simulink model "Lab3"  (R2023a)
settings: Solver=ode45  StartTime=0.0  StopTime=100  RelTol=1e-3
StopFcn:
  | % figure
  | % plot(20*log10(abs(fft(filter_out))));
undefined symbols (not defined in the file): xc7k325tfbg676
libraries: hdlBasic x35, vmcUtilities x1, dspsrcs4 x1
settings Model: Creator=scaffee  LastModifiedBy=robg
settings SolverCC: AlgebraicLoopSolver=TrustRegion
settings DataIOCC: LimitDataPoints=on  SaveFormat=Array  SignalLoggingSaveFormat=ModelDataLogs  ReturnWorkspaceOutputs=off
settings OptimizationCC: BlockReduction=off  BooleanDataType=off  LifeSpan=inf
settings DebuggingCC: SaveWithParameterizedLinksMsg=none  UnderspecifiedInitializationDetection=Classic  MergeDetectMultiDrivingBlocksExec=none  SignalResolutionControl=TryResolveAllWithWarning  MultiTaskDSMMsg=warning  MultiTaskCondExecSysMsg=none  UnconnectedInputMsg=warning  UnconnectedOutputMsg=warning  UnconnectedLineMsg=warning  AllowSymbolicDim=off  StateNameClashWarn=warning  SFUnexpectedBacktrackingDiag=warning  SFNoUnconditionalDefaultTransitionDiag=warning  ArithmeticOperatorsInVariantConditions=warning
settings HardwareCC: ProdBitPerPointer=32  ProdBitPerSizeT=32  ProdBitPerPtrDiffT=32  ProdLargestAtomicFloat=None  ProdIntDivRoundTo=Undefined  ProdEndianess=Unspecified  ProdWordSize=32  ProdHWDeviceType=32-bit Generic  TargetUnknown=on
settings ModelReferenceCC: EnableRefExpFcnMdlSchedulingChecks=on  PropagateSignalLabelsOutOfModel=off
settings SFSimCC: SimUseLocalCustomCode=off  CustomCodeUndefinedFunction=UseInterfaceOnly
settings RTWCC: RTWUseLocalCustomCode=off  DLArmComputeVersion=19.05
settings CodeAppCC: StateflowObjectComments=on
settings GRTTargetCC: TargetLangStandard=C89/C90 (ANSI)
settings ConfigComp: CovMetricSettings=dw  CovSaveCumulativeToWorkspaceVar=on  CovSaveSingleToWorkspaceVar=on  CovExternalEMLEnable=off

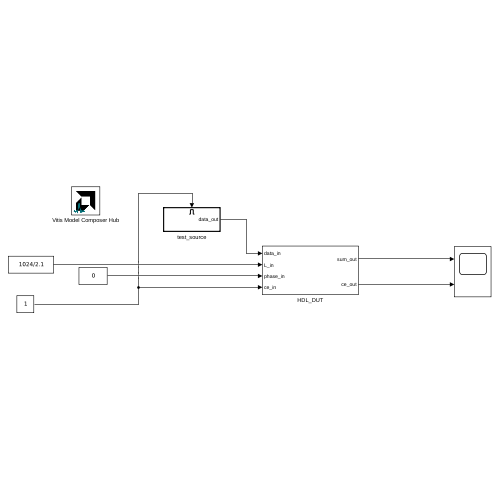
[thumbnail: Simulink's stored preview of the top-level diagram]
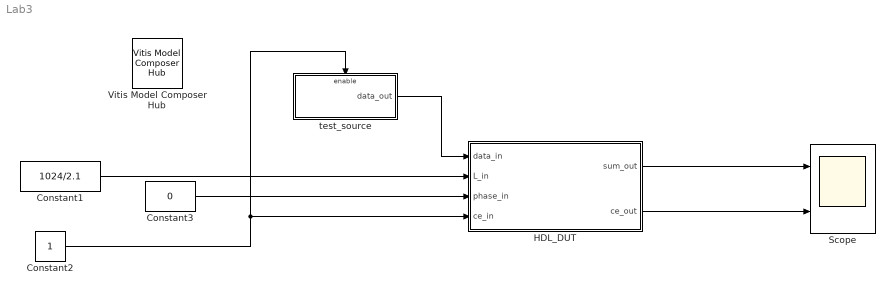
== system Lab3 ==
  Constant1 : Constant  Value=1024/2.1
  Constant2 : Constant
  Constant3 : Constant  Value=0
  HDL_DUT : Subsystem
  Scope : Scope  NumInputPorts=2
  Vitis Model Composer Hub : vmcUtilities/Vitis Model Composer Hub  Tag=genX  CodeGeneration=off  SubsystemName=HDL_DUT  StartColumn=1  NumberOfColumns=1  TargetDirectory=./code  exportDesign=off  analyzeDesign=off  validateDesignOnHw=off  ExportType=System Generator  IpVendor=xilinx.com  IpLibrary=hls  IpVersion=1.0  IpHWLanguage=Verilog  AieCompilerOptions={}  AieSimulatorOptions={}  CreateTestbench=off  TestbenchStackSize=10  RunRtlSim=off  RunCSim=off  RunAieSim=off  AieSimTimeout=50000  RunAieSimProfiling=off  LaunchVitisAnalyzer=off  PlotOutput=off  RunX86Sim=off  X86SimTimeout=10  GenHwImage=off  GenLibadfXo=on  GenHwValidationCode=off  PlatformType=Not Specified  HwSystemType=Baremetal  HwValidationTarget=hw  ProjDevice=xc7k325tfbg676-3  ProjDevicePart=xc7k325tfbg676-3  SamplePeriod=-1  ClockFrequency=200  DataPathParallelism=1  xilinxfamily=kintex7  part=xc7k325t  speed=-3  package=fbg676  directory=./netlist/ip/HDL_DUT/src  testbench=off  incr_netlist=off  synthesis_tool=Vivado  clock_wrapper=Clock Enables  dbl_ovrd=According to Block Masks  dcm_input_clock_period=10  sysclk_period=4  simulink_period=1  eval_field=0  LogFileName=''  NThreads=4
  test_source : Subsystem  TreatAsAtomicUnit=on
  wires:
  Constant2/1 -> HDL_DUT/4(ce_in), test_source/Enable
  test_source/1(data_out) -> HDL_DUT/1(data_in)
  Constant1/1 -> HDL_DUT/2(L_in)
  Constant3/1 -> HDL_DUT/3(phase_in)
  HDL_DUT/1(sum_out) -> Scope/1
  HDL_DUT/2(ce_out) -> Scope/2

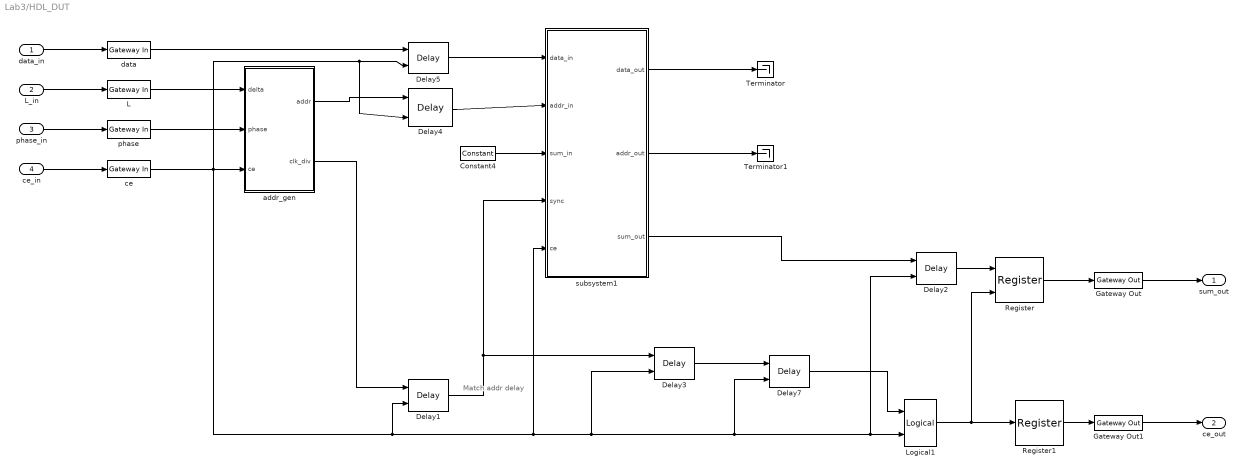
== system Lab3/HDL_DUT ==
  note: Match addr delay
  data_in : Inport
  L_in : Inport  Port=2
  phase_in : Inport  Port=3
  ce_in : Inport  Port=4
  Constant4 : hdlBasic/Constant  const=0  gui_display_data_type=Fixed-point  arith_type=Signed (2's comp)  n_bits=48  bin_pt=34  preci_type=Single  exp_width=8  frac_width=24  explicit_period=off  period=1  XmcBlockStatus=1  maskContainerNames=tabcontainer1  block_type=constant  block_config=sysgen:Constant_config
  Delay1 : hdlBasic/Delay  rst=off  en=on  latency=2  reg_retiming=on  XmcBlockStatus=1  maskContainerNames=group1  block_type=delay  block_config=sysgen:Delay_config
  Delay2 : hdlBasic/Delay  rst=off  en=on  latency=1  reg_retiming=on  XmcBlockStatus=1  maskContainerNames=group1  block_type=delay  block_config=sysgen:Delay_config
  Delay3 : hdlBasic/Delay  rst=off  en=on  latency=4  reg_retiming=on  XmcBlockStatus=1  maskContainerNames=group1  block_type=delay  block_config=sysgen:Delay_config
  Delay4 : hdlBasic/Delay  rst=off  en=on  latency=2  reg_retiming=on  XmcBlockStatus=1  maskContainerNames=group1  block_type=delay  block_config=sysgen:Delay_config
  Delay5 : hdlBasic/Delay  rst=off  en=on  latency=2  reg_retiming=on  XmcBlockStatus=1  maskContainerNames=group1  block_type=delay  block_config=sysgen:Delay_config
  Delay7 : hdlBasic/Delay  rst=off  en=on  latency=1  reg_retiming=on  XmcBlockStatus=1  maskContainerNames=group1  block_type=delay  block_config=sysgen:Delay_config
  Gateway Out : hdlBasic/Gateway Out  inherit_from_input=off  hdl_port=on  rows=1  columns=1  UseAsDAC=off  DACChannel='1'  interface=None  automatic_assignment=on  address_offset=hex2dec('00')  intf_name=''  intf_description=''  timing_constraint=None  locs_specified=off  LOCs={}  io_standard={}  XmcBlockStatus=1  maskContainerNames=group4  block_type=gatewayout  block_config=sysgen:gateway_out_config  block_width_w=590  block_height_w=620  block_width=620  block_height=750
  Gateway Out1 : hdlBasic/Gateway Out  inherit_from_input=off  hdl_port=on  rows=1  columns=1  UseAsDAC=off  DACChannel='1'  interface=None  automatic_assignment=on  address_offset=hex2dec('00')  intf_name=''  intf_description=''  timing_constraint=None  locs_specified=off  LOCs={}  io_standard={}  XmcBlockStatus=1  maskContainerNames=group4  block_type=gatewayout  block_config=sysgen:gateway_out_config  block_width_w=590  block_height_w=620  block_width=620  block_height=750
  L : hdlBasic/Gateway In  gui_display_data_type=Fixed-point  arith_type=Unsigned  n_bits=32  bin_pt=21  preci_type=Single  exp_width=8  frac_width=24  rows=1  columns=1  quantization="Round  (unbiased: +/- Inf)"  overflow=Saturate  period=1  UseAsADC=off  ADCChannel='1'  interface=None  automatic_assignment=on  address_offset=hex2dec('00')  intf_name=''  intf_description=''  default_value=0  timing_constraint=None  locs_specified=off  LOCs={}  io_standard={}  inherit_from_input=off  hdl_port=on  XmcBlockStatus=1  maskContainerNames=group4  block_type=gatewayin  block_config=sysgen:gateway_in_config  block_width_w=590  block_height_w=620  block_width=640  block_height=850
  Logical1 : hdlBasic/Logical  logical_function=AND  inputs=2  en=off  latency=0  precision=Full  arith_type=Unsigned  n_bits=8  bin_pt=2  align_bp=on  overflow=[]  quantization=[]  XmcBlockStatus=1  maskContainerNames=tabcontainer1  block_type=logical  block_config=sysgen:Logical_config
  Register : hdlBasic/Register  init=0  rst=off  en=on  XmcBlockStatus=1  maskContainerNames=tabcontainer1  block_type=register  block_config=sysgen:Register_config
  Register1 : hdlBasic/Register  init=0  rst=off  en=off  XmcBlockStatus=1  maskContainerNames=tabcontainer1  block_type=register  block_config=sysgen:Register_config
  Terminator : Terminator
  Terminator1 : Terminator
  addr_gen : Subsystem
  ce : hdlBasic/Gateway In  gui_display_data_type=Boolean  arith_type=Boolean  n_bits=8  bin_pt=0  preci_type=Single  exp_width=8  frac_width=24  rows=1  columns=1  quantization="Round  (unbiased: +/- Inf)"  overflow=Saturate  period=1  UseAsADC=off  ADCChannel='1'  interface=None  automatic_assignment=on  address_offset=hex2dec('00')  intf_name=''  intf_description=''  default_value=0  timing_constraint=None  locs_specified=off  LOCs={}  io_standard={}  inherit_from_input=off  hdl_port=on  XmcBlockStatus=1  maskContainerNames=group4  block_type=gatewayin  block_config=sysgen:gateway_in_config  block_width_w=590  block_height_w=620  block_width=640  block_height=850
  data : hdlBasic/Gateway In  gui_display_data_type=Fixed-point  arith_type=Signed (2's comp)  n_bits=18  bin_pt=17  preci_type=Single  exp_width=8  frac_width=24  rows=1  columns=1  quantization="Round  (unbiased: +/- Inf)"  overflow=Saturate  period=1  UseAsADC=off  ADCChannel='1'  interface=None  automatic_assignment=on  address_offset=hex2dec('00')  intf_name=''  intf_description=''  default_value=0  timing_constraint=None  locs_specified=off  LOCs={}  io_standard={}  inherit_from_input=off  hdl_port=on  XmcBlockStatus=1  maskContainerNames=group4  block_type=gatewayin  block_config=sysgen:gateway_in_config  block_width_w=590  block_height_w=620  block_width=640  block_height=850
  phase : hdlBasic/Gateway In  gui_display_data_type=Fixed-point  arith_type=Unsigned  n_bits=10  bin_pt=0  preci_type=Single  exp_width=8  frac_width=24  rows=1  columns=1  quantization="Round  (unbiased: +/- Inf)"  overflow=Saturate  period=1  UseAsADC=off  ADCChannel='1'  interface=None  automatic_assignment=on  address_offset=hex2dec('00')  intf_name=''  intf_description=''  default_value=0  timing_constraint=None  locs_specified=off  LOCs={}  io_standard={}  inherit_from_input=off  hdl_port=on  XmcBlockStatus=1  maskContainerNames=group4  block_type=gatewayin  block_config=sysgen:gateway_in_config  block_width_w=590  block_height_w=620  block_width=640  block_height=850
  subsystem1 : Subsystem  mask{hhpoly1=8}
      mask prompts: hhpoly1 "Filter coefficients column?"
  sum_out : Outport
  ce_out : Outport  Port=2
  wires:
  addr_gen/1(addr) -> Delay4/1
  subsystem1/3(sum_out) -> Delay2/1
  Register1/1 -> Gateway Out1/1
  Delay2/1 -> Register/1
  Delay4/1 -> subsystem1/2(addr_in)
  Gateway Out/1 -> sum_out/1
  Delay5/1 -> subsystem1/1(data_in)
  addr_gen/2(clk_div) -> Delay1/1
  Gateway Out1/1 -> ce_out/1
  phase/1 -> addr_gen/2(phase)
  ce_in/1 -> ce/1
  Delay7/1 -> Logical1/1
  data/1 -> Delay5/1
  L_in/1 -> L/1
  phase_in/1 -> phase/1
  Logical1/1 -> Register/2, Register1/1
  Constant4/1 -> subsystem1/3(sum_in)
  subsystem1/2(addr_out) -> Terminator1/1
  subsystem1/1(data_out) -> Terminator/1
  Delay1/1 -> subsystem1/4(sync), Delay3/1
  Register/1 -> Gateway Out/1
  ce/1 -> Delay4/2, Delay5/2, addr_gen/3(ce), Delay1/2, subsystem1/5(ce), Delay3/2, Delay7/2, Delay2/2, Logical1/2
  data_in/1 -> data/1
  L/1 -> addr_gen/1(delta)
  Delay3/1 -> Delay7/1

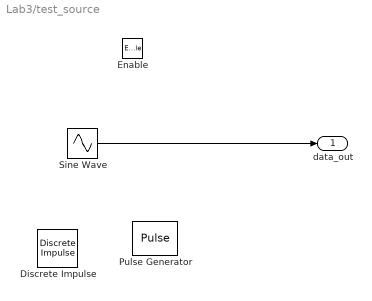
== system Lab3/test_source ==
  Enable : EnablePort
  Discrete Impulse : dspsrcs4/Discrete  Impulse  Delay=101  SampleTime=1  FrameSample=1  OutputFrames=on  dataType=double  isSigned=on  wordLen=16  udDataType=sfix(16)  fracBitsMode=Best precision  numFracBits=15  OutDataTypeStr=double  LastOutDataTypeStr=double
  Pulse Generator : DiscretePulseGenerator  Period=2048  PulseWidth=512
  Sine Wave : Sin  SineType=Sample based  Samples=3*1000  SampleTime=1
  data_out : Outport  VectorParamsAs1DForOutWhenUnconnected=off
  wires:
  Sine Wave/1 -> data_out/1

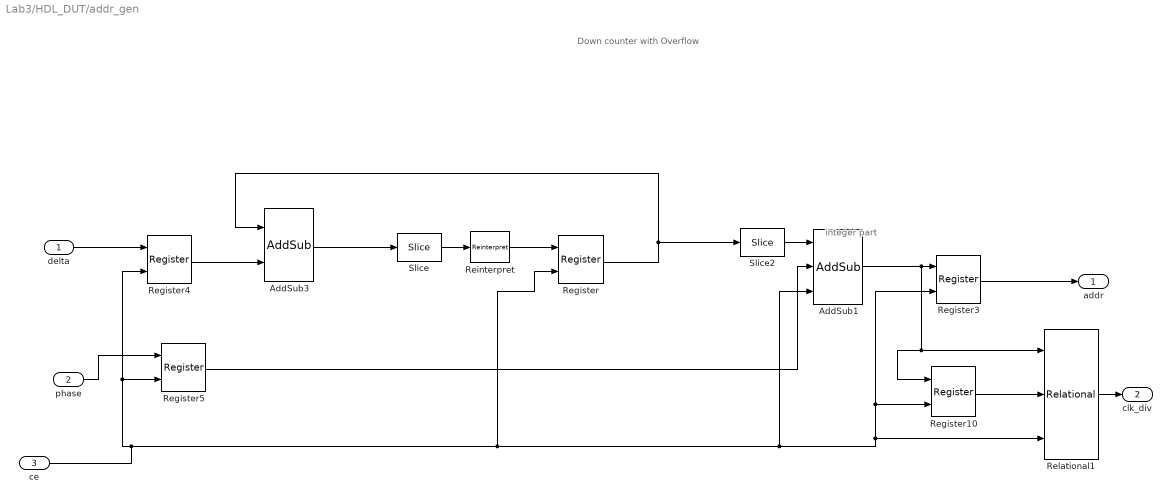
== system Lab3/HDL_DUT/addr_gen ==
  note: Down counter with Overflow
  note: integer part
  delta : Inport
  phase : Inport  Port=2
  ce : Inport  Port=3
  AddSub1 : hdlBasic/AddSub  mode=Addition  use_carryin=off  use_carryout=off  en=on  latency=1  precision=User Defined  arith_type=Unsigned  n_bits=10  bin_pt=0  quantization=Truncate  overflow=Wrap  use_behavioral_HDL=on  hw_selection=Fabric  pipelined=off  use_rpm=on  XmcBlockStatus=1  maskContainerNames=tabcontainer1  block_type=addsub  block_config=sysgen:Addsub_config
  AddSub3 : hdlBasic/AddSub  mode=Subtraction  use_carryin=off  use_carryout=off  en=off  latency=0  precision=User Defined  arith_type=Unsigned  n_bits=33  bin_pt=22  quantization="Round  (unbiased: +/- Inf)"  overflow=Wrap  use_behavioral_HDL=off  hw_selection=Fabric  pipelined=off  use_rpm=on  XmcBlockStatus=1  maskContainerNames=tabcontainer1  block_type=addsub  block_config=sysgen:Addsub_config
  Register{,3..5,10} (5 alike) : hdlBasic/Register  init=0  rst=off  en=on  XmcBlockStatus=1  maskContainerNames=tabcontainer1  block_type=register  block_config=sysgen:Register_config
  Reinterpret : hdlBasic/Reinterpret  force_arith_type=on  arith_type=Unsigned  force_bin_pt=on  bin_pt=22  XmcBlockStatus=1  maskContainerNames=group1  block_type=cast  block_config=sysgen:Reinterpret_config
  Relational1 : hdlBasic/Relational  mode=a>=b  op_type=Bool  en=on  latency=1  XmcBlockStatus=1  maskContainerNames=tabcontainer1  block_type=relational  block_config=sysgen:Relational_config
  Slice : hdlBasic/Slice  nbits=32  boolean_output=off  mode=Lower Bit Location + Width  bit1=1  base1=MSB of Input  bit0=0  base0=LSB of Input  XmcBlockStatus=1  maskContainerNames=group1  block_type=slice  block_config=sysgen:Slice_config
  Slice2 : hdlBasic/Slice  nbits=10  boolean_output=off  mode=Upper Bit Location + Width  bit1=0  base1=MSB of Input  bit0=0  base0=LSB of Input  XmcBlockStatus=1  maskContainerNames=group1  block_type=slice  block_config=sysgen:Slice_config
  addr : Outport  VectorParamsAs1DForOutWhenUnconnected=off
  clk_div : Outport  Port=2  VectorParamsAs1DForOutWhenUnconnected=off
  wires:
  Register/1 -> AddSub3/1, Slice2/1
  AddSub3/1 -> Slice/1
  Slice/1 -> Reinterpret/1
  Reinterpret/1 -> Register/1
  Slice2/1 -> AddSub1/1
  Register4/1 -> AddSub3/2
  delta/1 -> Register4/1
  phase/1 -> Register5/1
  Register5/1 -> AddSub1/2
  Register3/1 -> addr/1
  Register10/1 -> Relational1/2
  AddSub1/1 -> Relational1/1, Register10/1, Register3/1
  ce/1 -> Register3/2, Register10/2, Relational1/3, AddSub1/3, Register/2, Register4/2, Register5/2
  Relational1/1 -> clk_div/1

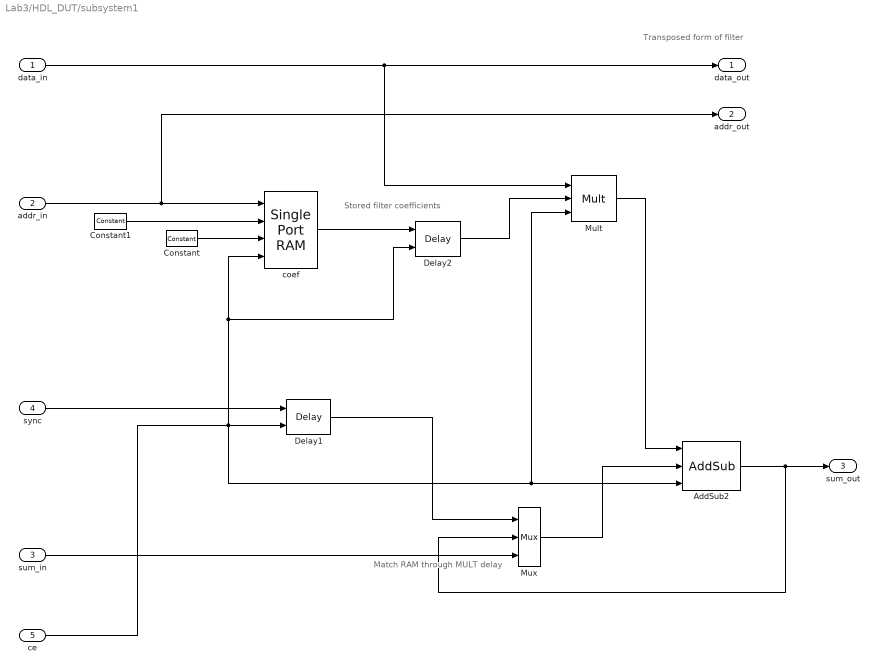
== system Lab3/HDL_DUT/subsystem1 ==
  note: Transposed form of filter
  note: Match RAM through MULT delay
  note: Stored filter coefficients
  data_in : Inport
  addr_in : Inport  Port=2
  sum_in : Inport  Port=3
  sync : Inport  Port=4
  ce : Inport  Port=5
  AddSub2 : hdlBasic/AddSub  mode=Addition  use_carryin=off  use_carryout=off  en=on  latency=1  precision=User Defined  arith_type="Signed  (2's comp)"  n_bits=48  bin_pt=34  quantization=Truncate  overflow=Wrap  use_behavioral_HDL=off  hw_selection=Fabric  pipelined=off  use_rpm=on  XmcBlockStatus=1  maskContainerNames=tabcontainer1  block_type=addsub  block_config=sysgen:Addsub_config
  Constant : hdlBasic/Constant  const=0  gui_display_data_type=Boolean  arith_type=Boolean  n_bits=1  bin_pt=0  preci_type=Single  exp_width=8  frac_width=24  explicit_period=off  period=1  XmcBlockStatus=1  maskContainerNames=tabcontainer1  block_type=constant  block_config=sysgen:Constant_config
  Constant1 : hdlBasic/Constant  const=0  gui_display_data_type=Fixed-point  arith_type=Signed (2's comp)  n_bits=18  bin_pt=17  preci_type=Single  exp_width=8  frac_width=24  explicit_period=off  period=1  XmcBlockStatus=1  maskContainerNames=tabcontainer1  block_type=constant  block_config=sysgen:Constant_config
  Delay1 : hdlBasic/Delay  rst=off  en=on  latency=4  reg_retiming=on  XmcBlockStatus=1  maskContainerNames=group1  block_type=delay  block_config=sysgen:Delay_config
  Delay2 : hdlBasic/Delay  rst=off  en=on  latency=1  reg_retiming=on  XmcBlockStatus=1  maskContainerNames=group1  block_type=delay  block_config=sysgen:Delay_config
  Mult : hdlBasic/Mult  precision=Full  arith_type="Signed  (2's comp)"  n_bits=36  bin_pt=34  quantization=Truncate  overflow=Wrap  en=on  latency=1  opt_float=off  fp_mult_usage=No Usage  use_behavioral_HDL=on  opt=Speed  use_embedded=on  optimum_pipeline=off  pipeline=off  use_rpm=on  placement_style=Rectangular shape  XmcBlockStatus=1  maskContainerNames=group1  block_type=mult  block_config=sysgen:Mult_config  block_width=598  block_height=876
  Mux : hdlBasic/Mux  inputs=2  en=off  latency=0  precision=Full  arith_type="Signed  (2's comp)"  n_bits=8  bin_pt=2  quantization=Truncate  overflow=Wrap  XmcBlockStatus=1  maskContainerNames=tabcontainer1  block_type=mux  block_config=sysgen:Mux_config
  coef : hdlBasic/Single Port RAM  depth=1024  initVector=1024  distributed_mem=Block RAM  write_mode=Read After Write  rst=off  init_reg=0  en=on  optimize_latency=on  latency=2  optimize=Speed  dbl_ovrd=off  simulation_type=fast_sim  XmcBlockStatus=1  maskContainerNames=tabcontainer1  block_type=spram  block_config=sysgen:SPRAM_config
  data_out : Outport  VectorParamsAs1DForOutWhenUnconnected=off
  addr_out : Outport  Port=2  VectorParamsAs1DForOutWhenUnconnected=off
  sum_out : Outport  Port=3  VectorParamsAs1DForOutWhenUnconnected=off
  wires:
  addr_in/1 -> addr_out/1, coef/1
  data_in/1 -> Mult/1, data_out/1
  sync/1 -> Delay1/1
  Constant/1 -> coef/3
  Constant1/1 -> coef/2
  coef/1 -> Delay2/1
  Delay2/1 -> Mult/2
  AddSub2/1 -> sum_out/1, Mux/2
  Mux/1 -> AddSub2/2
  sum_in/1 -> Mux/3
  Mult/1 -> AddSub2/1
  ce/1 -> AddSub2/3, Mult/3, Delay1/2, coef/4, Delay2/2
  Delay1/1 -> Mux/1
